simulink model "four_point_fft"  (R2018a)
settings: Solver=VariableStepAuto  StartTime=0.0  StopTime=10.0  RelTol=1e-3
undefined symbols (not defined in the file): j
settings Model: Creator=eechris  LastModifiedBy=eechris

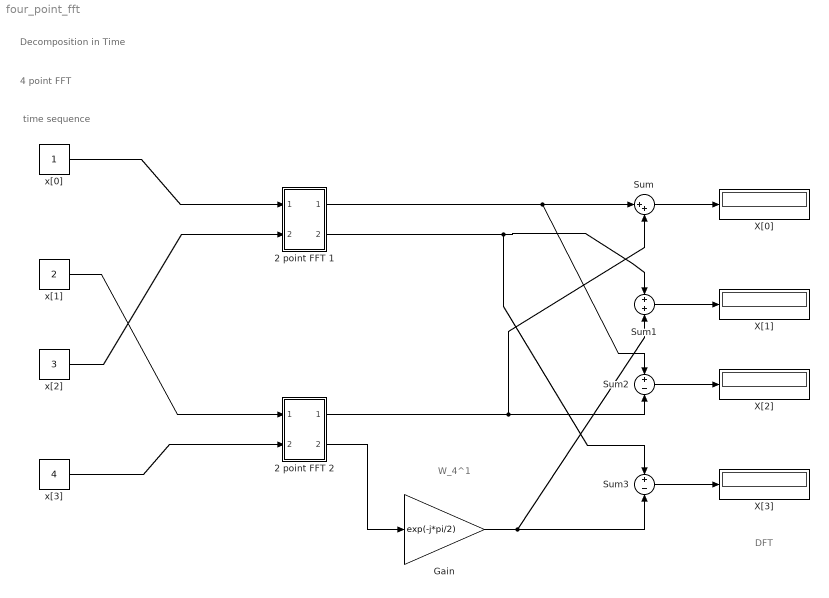
== system four_point_fft ==
  note: Decomposition in Time
  note: W_4^1
  note: time sequence
  note: DFT
  note: 4 point FFT
  2 point FFT 1 : Subsystem
  2 point FFT 2 : Subsystem
  Gain : Gain  Gain=exp(-j*pi/2)
  Sum : Sum  Inputs=|++
  Sum1 : Sum
  Sum2 : Sum  Inputs=+-
  Sum3 : Sum  Inputs=+-
  X[0] : Display
  X[1] : Display
  X[2] : Display
  X[3] : Display
  x[0] : Constant
  x[1] : Constant  Value=2
  x[2] : Constant  Value=3
  x[3] : Constant  Value=4
  wires:
  x[0]/1 -> 2 point FFT 1/1(In1)
  2 point FFT 1/1(Out1) -> Sum2/1, Sum/1
  2 point FFT 1/2(Out2) -> Sum1/1, Sum3/1
  x[3]/1 -> 2 point FFT 2/2(In2)
  2 point FFT 2/1(Out1) -> Sum2/2, Sum/2
  2 point FFT 2/2(Out2) -> Gain/1
  Sum/1 -> X[0]/1
  Sum1/1 -> X[1]/1
  Sum2/1 -> X[2]/1
  Sum3/1 -> X[3]/1
  Gain/1 -> Sum1/2, Sum3/2
  x[1]/1 -> 2 point FFT 2/1(In1)
  x[2]/1 -> 2 point FFT 1/2(In2)

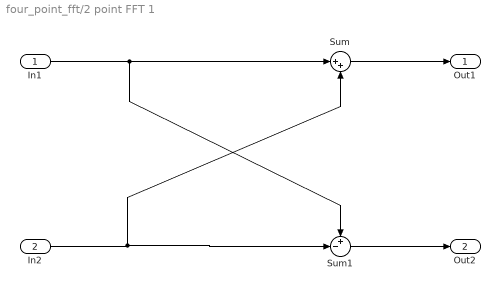
== system four_point_fft/2 point FFT 1 ==
  In1 : Inport
  In2 : Inport  Port=2
  Sum : Sum  Inputs=|++
  Sum1 : Sum  Inputs=+-|
  Out1 : Outport
  Out2 : Outport  Port=2
  wires:
  Sum/1 -> Out1/1
  In1/1 -> Sum1/1, Sum/1
  Sum1/1 -> Out2/1
  In2/1 -> Sum/2, Sum1/2

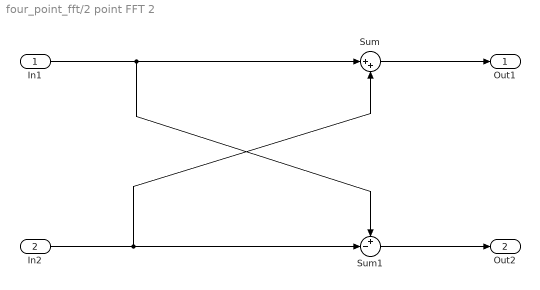
== system four_point_fft/2 point FFT 2 ==
  In1 : Inport
  In2 : Inport  Port=2
  Sum : Sum  Inputs=|++
  Sum1 : Sum  Inputs=+-|
  Out1 : Outport
  Out2 : Outport  Port=2
  wires:
  In2/1 -> Sum/2, Sum1/2
  Sum1/1 -> Out2/1
  In1/1 -> Sum/1, Sum1/1
  Sum/1 -> Out1/1
